simulink library "actuator_lib"  (Simulink 6.6)
libraries: actuator_S2_lib x2, actuator_T2_lib x1, simulink x1
settings Model: Creator=amurch  LastModifiedBy=amurch  ExtModeAutoUpdateStatusClock=off

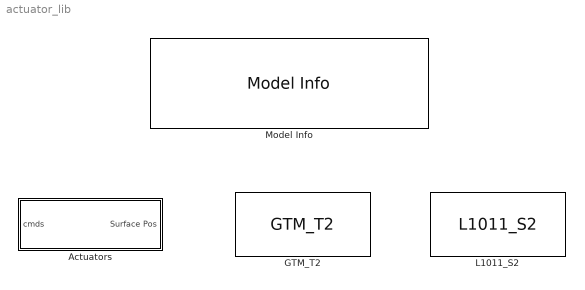
== system actuator_lib ==
  Actuators : Subsystem  BlockChoice=L1011_S2
      settings: TemplateBlock=self  MemberBlocks=GTM_T2,L1011_S2
  GTM_T2 : actuator_T2_lib/GTM_T2  SystemSampleTime=-1
  L1011_S2 : actuator_S2_lib/L1011_S2  SystemSampleTime=-1
  Model Info : simulink/Model-Wide Utilities/Model Info  SystemSampleTime=-1  InitialBlockCM=None  BlockCM=None  Frame=on  DisplayStringWithTags=|  HorizontalTextAlignment=Center  LeftAlignmentValue=0.5  SourceBlockDiagram=actuator_lib  TagMaxNumber=20
      | Actuator Library
      | %<ModelVersion>
      | Las modified by %<LastModifiedBy> on %<LastModificationDate>

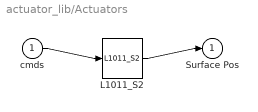
== system actuator_lib/Actuators ==
  cmds : Inport
  L1011_S2 : actuator_S2_lib/L1011_S2  SystemSampleTime=-1
  Surface Pos : Outport
  wires:
  cmds/1 -> L1011_S2/1
  L1011_S2/1 -> Surface Pos/1
